simulink model "Urban_Air_Mobility_v3"  (R2021a)
settings: Solver=ode4  StartTime=0.0  StopTime=50  FixedStep=0.01  RelTol=1e-3
model workspace (MAT data in the model file):
  op_trim2 : handle (value not decoded)
undefined symbols (not defined in the file or in its folder): BackProp, Earth, ForwProp, geo, initialise, mass, simsetup, WGS84
libraries: dspindex x6, aerolibactuator x4, sharedutil x3, simulink x3, aerolibasang x2, aerolibtransform2 x2, aerolibutil x2, shared6dof x1, aerolibatmos2 x1, sharedtransform x1, aerolibconvert2 x1
(part 2 of 3)

== system Urban_Air_Mobility_v3/Urban Air Vehicle Airframe Flight Dynamic Model/Lateral Directional Derivatives ==
  Mass (kg) : Inport
  Altitude (m) : Inport  Port=2
  Mach no. : Inport  Port=3
  CG (m) : Inport  Port=4
  CYb : Lookup_n-D  NumberOfTableDimensions=4  BreakpointsForDimension1=initialise.mass  BreakpointsForDimension2=initialise.Altitude  BreakpointsForDimension3=initialise.MLUT  BreakpointsForDimension4=initialise.CG  Table=initialise.CYb  InternalRulePriority=Speed  RndMeth=Simplest  InputSameDT=on
      settings: InputPortMap=u0,u1,u2,u3
  CYp : Lookup_n-D  NumberOfTableDimensions=4  BreakpointsForDimension1=initialise.mass  BreakpointsForDimension2=initialise.Altitude  BreakpointsForDimension3=initialise.MLUT  BreakpointsForDimension4=initialise.CG  Table=initialise.CYp  InternalRulePriority=Speed  RndMeth=Simplest  InputSameDT=on
      settings: InputPortMap=u0,u1,u2,u3
  CYr : Lookup_n-D  NumberOfTableDimensions=4  BreakpointsForDimension1=initialise.mass  BreakpointsForDimension2=initialise.Altitude  BreakpointsForDimension3=initialise.MLUT  BreakpointsForDimension4=initialise.CG  Table=initialise.CYr  InternalRulePriority=Speed  RndMeth=Simplest  InputSameDT=on
      settings: InputPortMap=u0,u1,u2,u3
  Clb : Lookup_n-D  NumberOfTableDimensions=4  BreakpointsForDimension1=initialise.mass  BreakpointsForDimension2=initialise.Altitude  BreakpointsForDimension3=initialise.MLUT  BreakpointsForDimension4=initialise.CG  Table=initialise.Clb  InternalRulePriority=Speed  RndMeth=Simplest  InputSameDT=on
      settings: InputPortMap=u0,u1,u2,u3
  Clp : Lookup_n-D  NumberOfTableDimensions=4  BreakpointsForDimension1=initialise.mass  BreakpointsForDimension2=initialise.Altitude  BreakpointsForDimension3=initialise.MLUT  BreakpointsForDimension4=initialise.CG  Table=initialise.Clp  InternalRulePriority=Speed  RndMeth=Simplest  InputSameDT=on
      settings: InputPortMap=u0,u1,u2,u3
  Clr : Lookup_n-D  NumberOfTableDimensions=4  BreakpointsForDimension1=initialise.mass  BreakpointsForDimension2=initialise.Altitude  BreakpointsForDimension3=initialise.MLUT  BreakpointsForDimension4=initialise.CG  Table=initialise.Clr  InternalRulePriority=Speed  RndMeth=Simplest  InputSameDT=on
      settings: InputPortMap=u0,u1,u2,u3
  "Cnb " : Lookup_n-D  NumberOfTableDimensions=4  BreakpointsForDimension1=initialise.mass  BreakpointsForDimension2=initialise.Altitude  BreakpointsForDimension3=initialise.MLUT  BreakpointsForDimension4=initialise.CG  Table=initialise.Cnb  InternalRulePriority=Speed  RndMeth=Simplest  InputSameDT=on
      settings: InputPortMap=u0,u1,u2,u3
  Cnp : Lookup_n-D  NumberOfTableDimensions=4  BreakpointsForDimension1=initialise.mass  BreakpointsForDimension2=initialise.Altitude  BreakpointsForDimension3=initialise.MLUT  BreakpointsForDimension4=initialise.CG  Table=initialise.Cnp  InternalRulePriority=Speed  RndMeth=Simplest  InputSameDT=on
      settings: InputPortMap=u0,u1,u2,u3
  Cnr : Lookup_n-D  NumberOfTableDimensions=4  BreakpointsForDimension1=initialise.mass  BreakpointsForDimension2=initialise.Altitude  BreakpointsForDimension3=initialise.MLUT  BreakpointsForDimension4=initialise.CG  Table=initialise.Cnr  InternalRulePriority=Speed  RndMeth=Simplest  InputSameDT=on
      settings: InputPortMap=u0,u1,u2,u3
  Cn_p : Outport  VectorParamsAs1DForOutWhenUnconnected=off
  Cn_r : Outport  Port=2  VectorParamsAs1DForOutWhenUnconnected=off
  Cl_p : Outport  Port=3  VectorParamsAs1DForOutWhenUnconnected=off
  Cl_r : Outport  Port=4  VectorParamsAs1DForOutWhenUnconnected=off
  CY_p : Outport  Port=5  VectorParamsAs1DForOutWhenUnconnected=off
  CY_r : Outport  Port=6  VectorParamsAs1DForOutWhenUnconnected=off
  CY_b : Outport  Port=7  VectorParamsAs1DForOutWhenUnconnected=off
  Cl_b : Outport  Port=8  VectorParamsAs1DForOutWhenUnconnected=off
  Cn_b : Outport  Port=9
  wires:
  CG (m)/1 -> Clb/4, CYb/4, "Cnb "/4, CYr/4, CYp/4, Clr/4, Clp/4, Cnr/4, Cnp/4
  Mass (kg)/1 -> Clb/1, CYb/1, "Cnb "/1, CYr/1, CYp/1, Clr/1, Clp/1, Cnr/1, Cnp/1
  Clp/1 -> Cl_p/1
  Cnr/1 -> Cn_r/1
  Cnp/1 -> Cn_p/1
  Mach no./1 -> Clb/3, CYb/3, "Cnb "/3, CYr/3, CYp/3, Clr/3, Clp/3, Cnr/3, Cnp/3
  Clr/1 -> Cl_r/1
  CYr/1 -> CY_r/1
  CYp/1 -> CY_p/1
  CYb/1 -> CY_b/1
  Clb/1 -> Cl_b/1
  Altitude (m)/1 -> Clb/2, CYb/2, "Cnb "/2, CYr/2, CYp/2, Clr/2, Clp/2, Cnr/2, Cnp/2
  "Cnb "/1 -> Cn_b/1

== system Urban_Air_Mobility_v3/Urban Air Vehicle Airframe Flight Dynamic Model/Longitudinal Derivatives ==
  Mass (kg) : Inport
  Altitude (m) : Inport  Port=2
  Mach no. : Inport  Port=3
  CG (m) : Inport  Port=4
  CLalpha : Lookup_n-D  NumberOfTableDimensions=4  BreakpointsForDimension1=initialise.mass  BreakpointsForDimension2=initialise.Altitude  BreakpointsForDimension3=initialise.MLUT  BreakpointsForDimension4=initialise.CG  Table=initialise.CLa  InternalRulePriority=Speed  RndMeth=Simplest  InputSameDT=on
      settings: InputPortMap=u0,u1,u2,u3
  CLq : Lookup_n-D  NumberOfTableDimensions=4  BreakpointsForDimension1=initialise.mass  BreakpointsForDimension2=initialise.Altitude  BreakpointsForDimension3=initialise.MLUT  BreakpointsForDimension4=initialise.CG  Table=initialise.CLq  InternalRulePriority=Speed  RndMeth=Simplest  InputSameDT=on
      settings: InputPortMap=u0,u1,u2,u3
  Cmalpha : Lookup_n-D  NumberOfTableDimensions=4  BreakpointsForDimension1=initialise.mass  BreakpointsForDimension2=initialise.Altitude  BreakpointsForDimension3=initialise.MLUT  BreakpointsForDimension4=initialise.CG  Table=initialise.Cma  InternalRulePriority=Speed  RndMeth=Simplest  InputSameDT=on
      settings: InputPortMap=u0,u1,u2,u3
  Cmq : Lookup_n-D  NumberOfTableDimensions=4  BreakpointsForDimension1=initialise.mass  BreakpointsForDimension2=initialise.Altitude  BreakpointsForDimension3=initialise.MLUT  BreakpointsForDimension4=initialise.CG  Table=initialise.Cmq  InternalRulePriority=Speed  RndMeth=Simplest  InputSameDT=on
      settings: InputPortMap=u0,u1,u2,u3
  CL_alpha : Outport  VectorParamsAs1DForOutWhenUnconnected=off
  CL_q : Outport  Port=2  VectorParamsAs1DForOutWhenUnconnected=off
  Cm_alpha : Outport  Port=3  VectorParamsAs1DForOutWhenUnconnected=off
  Cm_q : Outport  Port=4  VectorParamsAs1DForOutWhenUnconnected=off
  wires:
  CG (m)/1 -> Cmq/4, Cmalpha/4, CLq/4, CLalpha/4
  Mass (kg)/1 -> Cmq/1, Cmalpha/1, CLq/1, CLalpha/1
  Cmalpha/1 -> Cm_alpha/1
  CLq/1 -> CL_q/1
  CLalpha/1 -> CL_alpha/1
  Mach no./1 -> Cmq/3, Cmalpha/3, CLq/3, CLalpha/3
  Cmq/1 -> Cm_q/1
  Altitude (m)/1 -> Cmq/2, Cmalpha/2, CLq/2, CLalpha/2

== system Urban_Air_Mobility_v3/Urban Air Vehicle Airframe Flight Dynamic Model/Zero conditions ==
  Mass (kg) : Inport
  Altitude (m) : Inport  Port=2
  Mach no. : Inport  Port=3
  Re : Inport  Port=4
  CG (m) : Inport  Port=5
  Drag Coefficient CD0 : Lookup_n-D  BreakpointsForDimension1=initialise.Re_range  BreakpointsForDimension2=initialise.Mach_range  BreakpointsForDimension3=initialise.MLUT  BreakpointsForDimension4=initialise.CG  Table=initialise.CD0  InternalRulePriority=Speed  RndMeth=Simplest  InputSameDT=on
      settings: InputPortMap=u0,u1
  Drag Coefficient CM : Lookup_n-D  NumberOfTableDimensions=4  BreakpointsForDimension1=initialise.mass  BreakpointsForDimension2=initialise.Altitude  BreakpointsForDimension3=initialise.MLUT  BreakpointsForDimension4=initialise.CG  Table=initialise.Cm0  InternalRulePriority=Speed  RndMeth=Simplest  InputSameDT=on
      settings: InputPortMap=u0,u1,u2,u3
  Lift Coefficient CL : Lookup_n-D  NumberOfTableDimensions=4  BreakpointsForDimension1=initialise.mass  BreakpointsForDimension2=initialise.Altitude  BreakpointsForDimension3=initialise.MLUT  BreakpointsForDimension4=initialise.CG  Table=initialise.CL0  InternalRulePriority=Speed  RndMeth=Simplest  InputSameDT=on
      settings: InputPortMap=u0,u1,u2,u3
  CL0 : Outport  VectorParamsAs1DForOutWhenUnconnected=off
  CD0 : Outport  Port=2  VectorParamsAs1DForOutWhenUnconnected=off
  CM0 : Outport  Port=3  VectorParamsAs1DForOutWhenUnconnected=off
  wires:
  CG (m)/1 -> Drag Coefficient CM/4, Lift Coefficient CL/4
  Mass (kg)/1 -> Drag Coefficient CM/1, Lift Coefficient CL/1
  Drag Coefficient CD0/1 -> CD0/1
  Lift Coefficient CL/1 -> CL0/1
  Mach no./1 -> Drag Coefficient CM/3, Drag Coefficient CD0/2, Lift Coefficient CL/3
  Altitude (m)/1 -> Drag Coefficient CM/2, Lift Coefficient CL/2
  Drag Coefficient CM/1 -> CM0/1
  Re/1 -> Drag Coefficient CD0/1

== system Urban_Air_Mobility_v3/Urban Air Vehicle Airframe Flight Dynamic Model/Forces and Moments calculation/Ground Effect  ==
  h_above_ground : Inport
  <q_dyn (Pa)> : Inport  Port=2
  CL_alpha : Inport  Port=3
  Drag : Inport  Port=4
  Lift : Inport  Port=5
  CL_dF : Inport  Port=6
  Cm_dF : Inport  Port=7
  Flap : Inport  Port=8
  VTAS : Inport  Port=9
  Enable : EnablePort  StatesWhenEnabling=reset
  Constant3 : Constant  Value=geo.mac_w
  Constant5 : Constant  Value=geo.b_fus+geo.b_w
  Constant6 : Constant  Value=geo.b_fus+geo.b_w
  Constant7 : Constant  Value=geo.S_w
  Constant8 : Constant  Value=geo.S_w
  Divide : Product  Inputs=*/
  Ground : Ground
  MATLAB Function1 : MATLAB Function  TreatAsAtomicUnit=on
  Square : Math  Operator=square  SignedPower=on  SaturateOnIntegerOverflow=on
  "Delta_lift " : Outport  OutputWhenDisabled=reset  InitialOutput=[0]  VectorParamsAs1DForOutWhenUnconnected=off
  Delta_drag : Outport  Port=2  OutputWhenDisabled=reset  InitialOutput=[0]  VectorParamsAs1DForOutWhenUnconnected=off
  Delta_CL : Outport  Port=3  OutputWhenDisabled=reset  InitialOutput=[0]  VectorParamsAs1DForOutWhenUnconnected=off
  "Delta_CD " : Outport  Port=4  OutputWhenDisabled=reset  InitialOutput=[0]  VectorParamsAs1DForOutWhenUnconnected=off
  wires:
  Constant8/1 -> MATLAB Function1/13(S_ref)
  MATLAB Function1/4(delta_Drag) -> Delta_drag/1
  MATLAB Function1/3(delta_Lift) -> "Delta_lift "/1
  Square/1 -> Divide/1
  Constant7/1 -> Divide/2
  Constant6/1 -> Square/1
  Divide/1 -> [C]
  CL_dF/1 -> MATLAB Function1/8(CL_dF)
  Lift/1 -> MATLAB Function1/7(Lift)
  CL_alpha/1 -> MATLAB Function1/1(lift_curve_slope)
  Constant3/1 -> MATLAB Function1/3(c_bar)
  h_above_ground/1 -> MATLAB Function1/2(height_above_ground)
  Cm_dF/1 -> MATLAB Function1/9(Cm_dF)
  Ground/1 -> MATLAB Function1/11(wing_thickness)
  [C] -> MATLAB Function1/5(AR)
  Drag/1 -> MATLAB Function1/6(Drag)
  Constant5/1 -> MATLAB Function1/4(b)
  <q_dyn (Pa)>/1 -> MATLAB Function1/12(q_dyn)
  MATLAB Function1/1(delta_CL) -> Delta_CL/1
  MATLAB Function1/2(delta_CD) -> "Delta_CD "/1
  Flap/1 -> MATLAB Function1/10(Flap)
  VTAS/1 -> MATLAB Function1/14(VTAS)

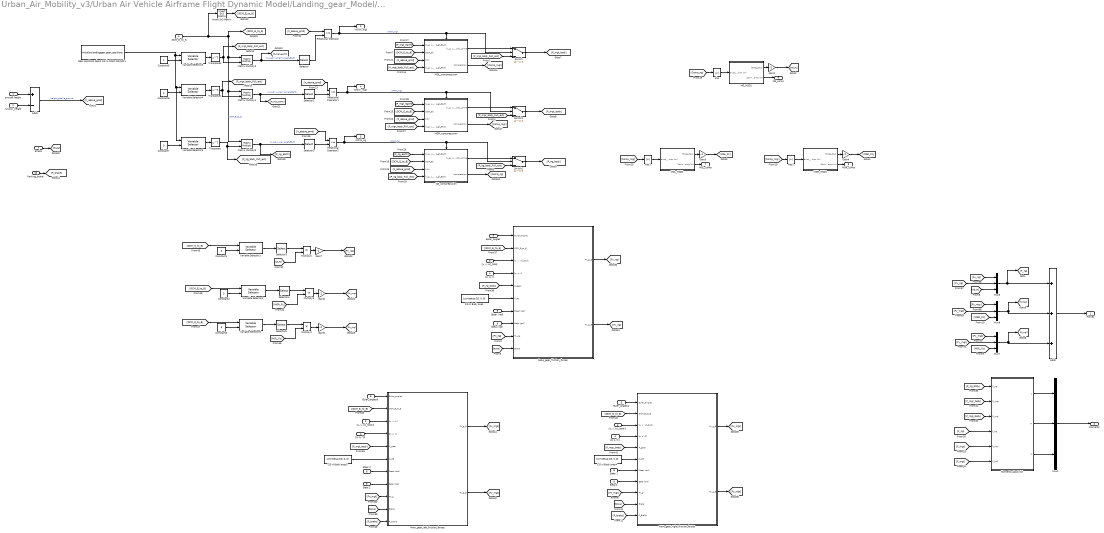
== system Urban_Air_Mobility_v3/Urban Air Vehicle Airframe Flight Dynamic Model/Landing_gear_Model/Landing Gear (with steer 4) ==
  aircraft height : Inport
  runway_height : Inport  Port=2
  DCM_B_to_E : Inport  Port=3
  "[p, q, r]" : Inport  Port=4
  "[u, v, w]_body" : Inport  Port=5
  Euler_angles : Inport  Port=6
  "Brake " : Inport  Port=7
  "Steer (rad) " : Inport  Port=8
  "Beta (rad) " : Inport  Port=9
  Parking_brake : Inport  Port=10
  Abs : Abs
  Abs1 : Abs
  Abs2 : Abs
  Add1 : Sum  Inputs=+-
  Add2 : Sum  Inputs=+++
  Beta 1 : InportShadow  Port=9
  Beta 2 : InportShadow  Port=9
  CG in Body axes : Constant  Value=[simsetup.CG, 0, 0]
  CG in Body axes3 : Constant  Value=[simsetup.CG, 0, 0]
  CG in Body axes4 : Constant  Value=[simsetup.CG, 0, 0]
  Constant{1..3,7} (4 alike) : Constant  Value=3
  Constant5 : Constant
  Constant6 : Constant  Value=2
  Euler_angles2 : InportShadow  Port=6
  Euler_angles6 : InportShadow  Port=6
  Gain{2..4,7..9} (6 alike) : Gain  Gain=-1
  Gear positions about CG (L.MG;R.MG;NG)1 : Constant  Value=initialise.landinggear.gear_positions
  Invert 3x3 Matrix : aerolibutil/Invert  3x3 Matrix
  MGL_MSD1 : Subsystem
  MGL_compresssion : Subsystem
  MGR_MSD1 : Subsystem
  MGR_compresssion : Subsystem
  Main_gear_left_friction_forces : Subsystem
  Main_gear_right_friction_forces : Subsystem
  Matrix Multiply3 : Product  Multiplication=Matrix(*)
  Matrix Multiply4 : Product  Multiplication=Matrix(*)
  Matrix Multiply5 : Product  Multiplication=Matrix(*)
  Moments about CG : MATLAB Function  TreatAsAtomicUnit=on
  Multiply2 : Product
  Multiply3 : Product
  Multiply4 : Product
  Mux{1,6..8} (4 alike) : Mux  Inputs=3
  NG_MSD1 : Subsystem
  NG_compresssion : Subsystem
  Nose_gear_friction_forces : Subsystem
  Relational Operator : RelationalOperator  Operator=<=  OutDataTypeStr=boolean  RndMeth=Simplest
  Relational Operator1 : RelationalOperator  Operator=<=  OutDataTypeStr=boolean  RndMeth=Simplest
  Relational Operator2 : RelationalOperator  Operator=<=  OutDataTypeStr=boolean  RndMeth=Simplest
  Selector{,1..5} (6 alike) : Selector  InputPortWidth=3  IndexOptions=Index vector (dialog)  Indices=3  OutputSizes=1
  Steer 1 : InportShadow  Port=8
  Steer 2 : InportShadow  Port=8
  Switch : Switch  Criteria=u2 ~= 0
  Switch1 : Switch  Criteria=u2 ~= 0
  Switch2 : Switch  Criteria=u2 ~= 0
  Transpose : Math  Operator=transpose  SignedPower=on  SaturateOnIntegerOverflow=on
  Transpose1 : Math  Operator=transpose  SignedPower=on  SaturateOnIntegerOverflow=on
  Transpose2 : Math  Operator=transpose  SignedPower=on  SaturateOnIntegerOverflow=on
  Variable Selector{1..6} (6 alike) : dspindex/Variable Selector  NumInputs=1  rowsOrCols=Rows  IdxMode=Variable  Elements=[1 3]  ZerOneIdxMode=One-based  errmode=Clip Index  FillMode=on  FillValues=0
  "[p, q, r]1" : InportShadow  Port=4
  "[p, q, r]2" : InportShadow  Port=4
  "[u, v, w]_body1" : InportShadow  Port=5
  "[u, v, w]_body2" : InportShadow  Port=5
  "Forces " : Outport  VectorParamsAs1DForOutWhenUnconnected=off
  Moments : Outport  Port=2  VectorParamsAs1DForOutWhenUnconnected=off
  WOW_mgl : Outport  Port=3  VectorParamsAs1DForOutWhenUnconnected=off
  WOW_mglr : Outport  Port=4  VectorParamsAs1DForOutWhenUnconnected=off
  "WOW_ng " : Outport  Port=5  VectorParamsAs1DForOutWhenUnconnected=off
  NG_comp : Outport  Port=6  VectorParamsAs1DForOutWhenUnconnected=off
  MGL_comp : Outport  Port=7  VectorParamsAs1DForOutWhenUnconnected=off
  MGR_comp : Outport  Port=8  VectorParamsAs1DForOutWhenUnconnected=off
  wires:
  Constant7/1 -> Variable Selector5/2
  [Fy_mgr] -> Mux8/2
  Selector2/1 -> Relational Operator2/2
  Selector/1 -> Relational Operator/2
  MGR_MSD1/1(Force_strut) -> Gain4/1
  DCM_B_to_E/1 -> Matrix Multiply5/1, Matrix Multiply4/1, Matrix Multiply3/1, [DCM_B_to_E], Invert 3x3 Matrix/1  "DCM_B_to_E"
  [Fx_mgr] -> Mux8/1
  MGL_compresssion/1("[x_g, y_g, z_g]_Body_prime") -> Switch/1
  Mux8/1 -> [F_mgr], Add2/2
  Relational Operator1/1 -> MGR_compresssion/Enable, Switch1/2, WOW_mglr/1  "WOW_mgr"
  [MGL_Fz] -> Mux7/3
  Gain4/1 -> [MGR_Fz]
  [P_mgl_body_Full_ext] -> MGL_compresssion/4("[x_g, y_g, z_g]_Body")
  [Comp_ng] -> Abs/1
  [Fy_ng] -> Mux6/2
  [DCM_E_to_B] -> NG_compresssion/2("DCM_eb ")
  [Fx_ng] -> Mux6/1
  [NG_Fz] -> Mux6/3
  [DCM_E_to_B] -> MGL_compresssion/2("DCM_eb ")
  [Comp_mgl] -> Abs1/1
  Matrix Multiply3/1 -> [P_mgl_earth], Selector/1  "[x_mgl, y_mgl, z_mgl]_Earth"
  Constant5/1 -> Variable Selector3/2
  MGL_MSD1/1(Force_strut) -> Gain3/1
  [MGR_Fz] -> Mux8/3
  [Fx_mgl] -> Mux7/1
  Add2/1 -> "Forces "/1
  Constant6/1 -> Variable Selector4/2
  [Fy_mgl] -> Mux7/2
  Variable Selector4/1 -> Transpose1/1
  Add1/1 -> [h_above_grnd]  "height_above_ground"
  Variable Selector3/1 -> Transpose2/1
  Variable Selector5/1 -> Transpose/1
  MGL_MSD1/2(Spring_comp (m)) -> MGL_comp/1
  Mux6/1 -> [F_ng], Add2/1
  [DCM_E_to_B] -> MGR_compresssion/2("DCM_eb ")
  Relational Operator/1 -> WOW_mgl/1, Switch/2, MGL_compresssion/Enable  "WOW_mgl"
  Mux7/1 -> [F_mgl], Add2/3
  Matrix Multiply4/1 -> [P_mgr_earth], Selector1/1  "[x_mgr, y_mgr, z_mgr]_Earth"
  Gain3/1 -> [MGL_Fz]
  [Comp_mgr] -> Abs2/1
  Selector1/1 -> Relational Operator1/2
  NG_MSD1/1(Force_strut) -> Gain2/1
  MGR_MSD1/2(Spring_comp (m)) -> MGR_comp/1
  [P_ng_body_Full_ext] -> NG_compresssion/4("[x_g, y_g, z_g]_Body")
  MGR_compresssion/2(compression) -> [Comp_mgr]
  NG_MSD1/2(Spring_comp (m)) -> NG_comp/1
  Gain2/1 -> [NG_Fz]
  Matrix Multiply5/1 -> [P_ng_earth], Selector2/1  "[x_ng, y_ng, z_ng]_Earth"
  NG_compresssion/2(compression) -> [Comp_ng]
  Relational Operator2/1 -> NG_compresssion/Enable, Switch2/2, "WOW_ng "/1  "WOW_ng"
  Invert 3x3 Matrix/1 -> [DCM_E_to_B]
  [P_mgr_body_Full_ext] -> MGR_compresssion/4("[x_g, y_g, z_g]_Body")
  NG_compresssion/1("[x_g, y_g, z_g]_Body_prime") -> Switch2/1
  runway_height/1 -> Add1/2
  MGR_compresssion/1("[x_g, y_g, z_g]_Body_prime") -> Switch1/1
  aircraft height/1 -> Add1/1
  [P_mgl_body_Full_ext] -> Switch/3
  Switch/1 -> [P_mgl_body]
  [P_mgr_body_Full_ext] -> Switch1/3
  Switch1/1 -> [P_mgr_body]
  [P_ng_body_Full_ext] -> Switch2/3
  Switch2/1 -> [P_ng_body]
  MGL_compresssion/2(compression) -> [Comp_mgl]
  Abs/1 -> NG_MSD1/1("axial_deflection (m) ")
  Abs1/1 -> MGL_MSD1/1("axial_deflection (m) ")
  Abs2/1 -> MGR_MSD1/1("axial_deflection (m) ")
  Transpose/1 -> [P_ng_body_Full_ext], Matrix Multiply5/2
  Transpose1/1 -> Matrix Multiply4/2, [P_mgr_body_Full_ext]
  Transpose2/1 -> Matrix Multiply3/2, [P_mgl_body_Full_ext]
  [h_above_grnd] -> MGL_compresssion/3("h-hr ")
  [h_above_grnd] -> MGR_compresssion/3("h-hr ")
  [h_above_grnd] -> NG_compresssion/3("h-hr ")
  [h_above_grnd] -> Relational Operator/1
  [h_above_grnd] -> Relational Operator1/1
  [h_above_grnd] -> Relational Operator2/1
  [P_mgl_earth] -> MGL_compresssion/1("[x_g, y_g, z_g]_Earth")
  [P_mgr_earth] -> MGR_compresssion/1("[x_g, y_g, z_g]_Earth")
  [P_ng_earth] -> NG_compresssion/1("[x_g, y_g, z_g]_Earth")
  [F_mgr] -> Moments about CG/5(F_mgr)
  [F_ng] -> Moments about CG/4(F_ng)
  Moments about CG/1(L) -> Mux1/1
  Mux1/1 -> Moments/1
  [F_mgl] -> Moments about CG/6(F_mgl)
  Moments about CG/3(N) -> Mux1/3
  [P_mgl_body] -> Moments about CG/3(P_mgl)
  Moments about CG/2(M) -> Mux1/2
  [P_ng_body] -> Moments about CG/1(P_ng)
  [P_mgr_body] -> Moments about CG/2(P_mgr)
  Gear positions about CG (L.MG;R.MG;NG)1/1 -> Variable Selector5/1, Variable Selector4/1, Variable Selector3/1
  [DCM_E_to_B] -> Variable Selector1/1
  Constant1/1 -> Variable Selector1/2
  Variable Selector1/1 -> Selector3/1
  Selector3/1 -> Multiply2/1
  [NG_Fz] -> Multiply2/2
  Multiply2/1 -> Gain7/1
  Multiply3/1 -> Gain8/1
  [MGR_Fz] -> Multiply3/2
  Selector4/1 -> Multiply3/1
  Variable Selector2/1 -> Selector4/1
  Constant2/1 -> Variable Selector2/2
  [DCM_E_to_B] -> Variable Selector2/1
  [DCM_E_to_B] -> Variable Selector6/1
  Constant3/1 -> Variable Selector6/2
  Variable Selector6/1 -> Selector5/1
  Selector5/1 -> Multiply4/1
  [MGL_Fz] -> Multiply4/2
  Multiply4/1 -> Gain9/1
  Gain7/1 -> [Fn_ng]
  Gain8/1 -> [Fn_mgr]
  Gain9/1 -> [Fn_mgl]
  "Brake "/1 -> [Brake]
  Parking_brake/1 -> [P_brake]
  Euler_angles/1 -> Nose_gear_friction_forces/1(Euler_angles)
  [DCM_B_to_E] -> Nose_gear_friction_forces/2(DCM_B_to_E)
  "[u, v, w]_body"/1 -> Nose_gear_friction_forces/3("[u, v, w]_body")
  "[p, q, r]"/1 -> Nose_gear_friction_forces/4("[p, q, r]")
  [P_ng_body] -> Nose_gear_friction_forces/5(P_gear)
  CG in Body axes/1 -> Nose_gear_friction_forces/6(P_cg)
  "Steer (rad) "/1 -> Nose_gear_friction_forces/7("Steer (rad) ")
  "Beta (rad) "/1 -> Nose_gear_friction_forces/8("Beta (rad) ")
  Nose_gear_friction_forces/1(Fx_g_E) -> [Fx_ng]
  Nose_gear_friction_forces/2(Fy_g_E) -> [Fy_ng]
  [Fn_ng] -> Nose_gear_friction_forces/9(Fn_ng)
  [Brake] -> Nose_gear_friction_forces/10("Brake ")
  [DCM_B_to_E] -> Main_gear_right_friction_forces/2(DCM_B_to_E)
  "[u, v, w]_body1"/1 -> Main_gear_right_friction_forces/3("[u, v, w]_body")
  "[p, q, r]1"/1 -> Main_gear_right_friction_forces/4("[p, q, r]]")
  [P_mgr_body] -> Main_gear_right_friction_forces/5(P_gear)
  Beta 1/1 -> Main_gear_right_friction_forces/8("Beta (rad) ")
  CG in Body axes4/1 -> Main_gear_right_friction_forces/6(P_CG)
  Steer 1/1 -> Main_gear_right_friction_forces/7("Steer (rad) ")
  Euler_angles2/1 -> Main_gear_right_friction_forces/1(Euler_angles)
  Main_gear_right_friction_forces/1(Fx_g_E) -> [Fx_mgr]
  Main_gear_right_friction_forces/2(Fy_g_E) -> [Fy_mgr]
  [Fn_mgr] -> Main_gear_right_friction_forces/9(Fn_g)
  [P_brake] -> Main_gear_right_friction_forces/11(P_Brake)
  [Brake] -> Main_gear_right_friction_forces/10(Brake)
  Euler_angles6/1 -> Main_gear_left_friction_forces/1(Euler_angles)
  [DCM_B_to_E] -> Main_gear_left_friction_forces/2(DCM_B_to_E)
  "[u, v, w]_body2"/1 -> Main_gear_left_friction_forces/3("[u, v, w]")
  "[p, q, r]2"/1 -> Main_gear_left_friction_forces/4("[p, q, r]")
  [P_mgl_body] -> Main_gear_left_friction_forces/5(P_gear)
  Beta 2/1 -> Main_gear_left_friction_forces/8("Beta (rad) ")
  CG in Body axes3/1 -> Main_gear_left_friction_forces/6(P_CG)
  Steer 2/1 -> Main_gear_left_friction_forces/7("Steer (rad) ")
  Main_gear_left_friction_forces/1(Fx_g_E) -> [Fx_mgl]
  Main_gear_left_friction_forces/2(Fy_g_E) -> [Fy_mgl]
  [Brake] -> Main_gear_left_friction_forces/10(Brake)
  [Fn_mgl] -> Main_gear_left_friction_forces/9(Fn_g)
  [P_brake] -> Main_gear_left_friction_forces/11(P_brake)

== system Urban_Air_Mobility_v3/Urban Air Vehicle Airframe Flight Dynamic Model/Landing_gear_Model/UC Aero Forces and Moments ==
  alpha : Inport
  Re : Inport  Port=2
  q_dyn : Inport  Port=3
  beta : Inport  Port=4
  flap_d : Inport  Port=5
  Angle Conversion : aerolibconvert2/Angle Conversion  IU=rad  OU=deg
  CD_main_landing_gear : Lookup_n-D  NumberOfTableDimensions=3  BreakpointsForDimension1=initialise.landinggear.aero.re  BreakpointsForDimension2=initialise.landinggear.aero.alpha  BreakpointsForDimension3=initialise.landinggear.aero.dflap  BreakpointsForDimension4=initialise.CG  Table=initialise.landinggear.aero.CD_maingear  InternalRulePriority=Speed  RndMeth=Simplest  InputSameDT=on
      settings: InputPortMap=u0,u1,u2
  CD_main_landing_gear to calculate side force : Lookup_n-D  NumberOfTableDimensions=3  BreakpointsForDimension1=initialise.landinggear.aero.re  BreakpointsForDimension2=initialise.landinggear.aero.alpha  BreakpointsForDimension3=initialise.landinggear.aero.dflap  BreakpointsForDimension4=initialise.CG  Table=initialise.landinggear.aero.CD_maingear  InternalRulePriority=Speed  RndMeth=Simplest  InputSameDT=on
      settings: InputPortMap=u0,u1,u2
  CD_nose_landing_gear : Lookup_n-D  BreakpointsForDimension1=initialise.landinggear.aero.re  BreakpointsForDimension2=initialise.landinggear.aero.alpha  BreakpointsForDimension3=initialise.landingear.dflap  BreakpointsForDimension4=initialise.CG  Table=initialise.landinggear.aero.CD_nosegear  InternalRulePriority=Speed  RndMeth=Simplest  InputSameDT=on
      settings: InputPortMap=u0,u1
  CD_nose_landing_gear to calculate side force : Lookup_n-D  BreakpointsForDimension1=initialise.landinggear.aero.re  BreakpointsForDimension2=initialise.landinggear.aero.alpha  BreakpointsForDimension3=initialise.landingear.dflap  BreakpointsForDimension4=initialise.CG  Table=initialise.landinggear.aero.CD_nosegear  InternalRulePriority=Speed  RndMeth=Simplest  InputSameDT=on
      settings: InputPortMap=u0,u1
  Constant1 : Constant  Value=0
  Gear positions about CG (L.MG;R.MG;NG)1 : Constant  Value=initialise.landinggear.gear_positions
  MATLAB Function : MATLAB Function  TreatAsAtomicUnit=on
  alpha1 : InportShadow
  z_main_landing_gear : Lookup_n-D  BreakpointsForDimension1=initialise.landinggear.aero.re  BreakpointsForDimension2=initialise.landinggear.aero.alpha  BreakpointsForDimension3=initialise.landingear.dflap  BreakpointsForDimension4=initialise.CG  Table=initialise.landinggear.aero.z_maingear  InternalRulePriority=Speed  RndMeth=Simplest  InputSameDT=on
      settings: InputPortMap=u0,u1
  z_nose_landing_gear : Lookup_n-D  BreakpointsForDimension1=initialise.landinggear.aero.re  BreakpointsForDimension2=initialise.landinggear.aero.alpha  BreakpointsForDimension3=initialise.landingear.dflap  BreakpointsForDimension4=initialise.CG  Table=initialise.landinggear.aero.z_nosegear  InternalRulePriority=Speed  RndMeth=Simplest  InputSameDT=on
      settings: InputPortMap=u0,u1
  UC_aero_forces : Outport  VectorParamsAs1DForOutWhenUnconnected=off
  wires:
  alpha/1 -> Angle Conversion/1  "alpha"
  Re/1 -> z_nose_landing_gear/1, z_main_landing_gear/1, CD_nose_landing_gear to calculate side force/1, CD_main_landing_gear to calculate side force/1, CD_nose_landing_gear/1, CD_main_landing_gear/1  "Re"
  q_dyn/1 -> MATLAB Function/1(q_dyn)  "q"
  flap_d/1 -> CD_main_landing_gear/3  "flap_d"
  z_main_landing_gear/1 -> MATLAB Function/8(z_mg)
  z_nose_landing_gear/1 -> MATLAB Function/9(z_ng)  "z_nosegear"
  Angle Conversion/1 -> z_nose_landing_gear/2, z_main_landing_gear/2, CD_main_landing_gear to calculate side force/3, CD_nose_landing_gear/2, CD_main_landing_gear/2
  Constant1/1 -> CD_nose_landing_gear to calculate side force/2, CD_main_landing_gear to calculate side force/2
  alpha1/1 -> MATLAB Function/2(alpha)  "alpha"
  beta/1 -> MATLAB Function/3(beta)  "beta"
  CD_main_landing_gear/1 -> MATLAB Function/4(CD_mg)
  CD_nose_landing_gear/1 -> MATLAB Function/5(CD_ng)
  CD_main_landing_gear to calculate side force/1 -> MATLAB Function/6(dfy_mg)
  CD_nose_landing_gear to calculate side force/1 -> MATLAB Function/7(dfy_ng)
  Gear positions about CG (L.MG;R.MG;NG)1/1 -> MATLAB Function/10(UC_pos)
  MATLAB Function/1(UC_forces) -> UC_aero_forces/1

== system Urban_Air_Mobility_v3/Urban Air Vehicle Airframe Flight Dynamic Model/Landing_gear_Model/Landing Gear (with steer 4)/MGL_MSD1 ==
  "axial_deflection (m) " : Inport
  Add : Sum
  Derivative : Derivative
  Stiffness : Gain  Gain=initialise.landinggear.K
  Viscous Damping : Gain  Gain=initialise.landinggear.C
  deflection_range_limit : Saturate  UpperLimit=1.5  LowerLimit=0
  Force_strut : Outport  VectorParamsAs1DForOutWhenUnconnected=off
  Spring_comp (m) : Outport  Port=2  VectorParamsAs1DForOutWhenUnconnected=off
  wires:
  "axial_deflection (m) "/1 -> deflection_range_limit/1
  Add/1 -> Force_strut/1  "Force_strut"
  Stiffness/1 -> Add/1
  deflection_range_limit/1 -> Spring_comp (m)/1, Derivative/1, Stiffness/1
  Derivative/1 -> Viscous Damping/1
  Viscous Damping/1 -> Add/2

== system Urban_Air_Mobility_v3/Urban Air Vehicle Airframe Flight Dynamic Model/Landing_gear_Model/Landing Gear (with steer 4)/MGL_compresssion ==
  "[x_g, y_g, z_g]_Earth" : Inport
  "DCM_eb " : Inport  Port=2
  "h-hr " : Inport  Port=3
  "[x_g, y_g, z_g]_Body" : Inport  Port=4
  Enable : EnablePort  StatesWhenEnabling=reset
  Demux : Demux  Outputs=3
  Matrix Multiply1 : Product  Multiplication=Matrix(*)
  Mux : Mux  Inputs=3
  Scope : Scope
  Selector3 : Selector  InputPortWidth=3  IndexOptions=Index vector (dialog)  Indices=3  OutputSizes=1
  Selector4 : Selector  InputPortWidth=3  IndexOptions=Index vector (dialog)  Indices=3  OutputSizes=1
  Subtract2 : Sum  Inputs=+-
  Terminator : Terminator
  "[x_g, y_g, z_g]_Body_prime" : Outport  VectorParamsAs1DForOutWhenUnconnected=off
  compression : Outport  Port=2  OutputWhenDisabled=reset  InitialOutput=[0]  VectorParamsAs1DForOutWhenUnconnected=off
  wires:
  "DCM_eb "/1 -> Matrix Multiply1/1
  Demux/2 -> Mux/2
  Demux/1 -> Mux/1
  Mux/1 -> Matrix Multiply1/2
  Matrix Multiply1/1 -> Selector3/1, "[x_g, y_g, z_g]_Body_prime"/1
  "[x_g, y_g, z_g]_Earth"/1 -> Demux/1
  Subtract2/1 -> Scope/1, compression/1  "comp"
  Selector3/1 -> Subtract2/2
  Selector4/1 -> Subtract2/1
  "[x_g, y_g, z_g]_Body"/1 -> Selector4/1
  Demux/3 -> Terminator/1
  "h-hr "/1 -> Mux/3

== system Urban_Air_Mobility_v3/Urban Air Vehicle Airframe Flight Dynamic Model/Landing_gear_Model/Landing Gear (with steer 4)/MGR_MSD1 ==
  "axial_deflection (m) " : Inport
  Add : Sum
  Derivative : Derivative
  Stiffness : Gain  Gain=initialise.landinggear.K
  Viscous Damping : Gain  Gain=initialise.landinggear.C
  deflection_range_limit : Saturate  UpperLimit=1.5  LowerLimit=0
  Force_strut : Outport  VectorParamsAs1DForOutWhenUnconnected=off
  Spring_comp (m) : Outport  Port=2  VectorParamsAs1DForOutWhenUnconnected=off
  wires:
  Viscous Damping/1 -> Add/2
  Derivative/1 -> Viscous Damping/1
  deflection_range_limit/1 -> Stiffness/1, Derivative/1, Spring_comp (m)/1
  Stiffness/1 -> Add/1
  Add/1 -> Force_strut/1  "Force_strut"
  "axial_deflection (m) "/1 -> deflection_range_limit/1

== system Urban_Air_Mobility_v3/Urban Air Vehicle Airframe Flight Dynamic Model/Landing_gear_Model/Landing Gear (with steer 4)/MGR_compresssion ==
  "[x_g, y_g, z_g]_Earth" : Inport
  "DCM_eb " : Inport  Port=2
  "h-hr " : Inport  Port=3
  "[x_g, y_g, z_g]_Body" : Inport  Port=4
  Enable : EnablePort  StatesWhenEnabling=reset
  Demux : Demux  Outputs=3
  Matrix Multiply1 : Product  Multiplication=Matrix(*)
  Mux : Mux  Inputs=3
  Selector3 : Selector  InputPortWidth=3  IndexOptions=Index vector (dialog)  Indices=3  OutputSizes=1
  Selector4 : Selector  InputPortWidth=3  IndexOptions=Index vector (dialog)  Indices=3  OutputSizes=1
  Subtract2 : Sum  Inputs=+-
  Terminator : Terminator
  "[x_g, y_g, z_g]_Body_prime" : Outport  VectorParamsAs1DForOutWhenUnconnected=off
  compression : Outport  Port=2  OutputWhenDisabled=reset  InitialOutput=[0]  VectorParamsAs1DForOutWhenUnconnected=off
  wires:
  "[x_g, y_g, z_g]_Body"/1 -> Selector4/1
  Selector4/1 -> Subtract2/1
  Selector3/1 -> Subtract2/2
  Subtract2/1 -> compression/1  "comp"
  "[x_g, y_g, z_g]_Earth"/1 -> Demux/1
  Matrix Multiply1/1 -> "[x_g, y_g, z_g]_Body_prime"/1, Selector3/1
  Mux/1 -> Matrix Multiply1/2
  Demux/1 -> Mux/1
  "h-hr "/1 -> Mux/3
  Demux/2 -> Mux/2
  Demux/3 -> Terminator/1
  "DCM_eb "/1 -> Matrix Multiply1/1

== system Urban_Air_Mobility_v3/Urban Air Vehicle Airframe Flight Dynamic Model/Landing_gear_Model/Landing Gear (with steer 4)/Main_gear_left_friction_forces ==
  Euler_angles : Inport
  DCM_B_to_E : Inport  Port=2
  "[u, v, w]" : Inport  Port=3
  "[p, q, r]" : Inport  Port=4
  P_gear : Inport  Port=5
  P_CG : Inport  Port=6
  "Steer (rad) " : Inport  Port=7
  "Beta (rad) " : Inport  Port=8
  Fn_g : Inport  Port=9
  Brake : Inport  Port=10
  P_brake : Inport  Port=11
  Euler_angles1 : InportShadow
  GP to Earth axes 2 : Subsystem
  MGL_friction_forces : Subsystem
  Velocity at MGL in ground path : Subsystem
  Fx_g_E : Outport  VectorParamsAs1DForOutWhenUnconnected=off
  Fy_g_E : Outport  Port=2  VectorParamsAs1DForOutWhenUnconnected=off
  wires:
  Velocity at MGL in ground path/2(v_g_gp) -> [v_mgl_gp]
  GP to Earth axes 2/2(Fy_g_E) -> Fy_g_E/1
  Brake/1 -> MGL_friction_forces/4(Brake)
  Velocity at MGL in ground path/1(u_g_gp) -> [u_mgl_gp]
  [F_long_mgl] -> GP to Earth axes 2/2(F_long_g)
  Euler_angles1/1 -> Velocity at MGL in ground path/6(Euler)
  [v_mgl_gp] -> MGL_friction_forces/3(v_gp)
  MGL_friction_forces/1(F_g_long) -> [F_long_mgl]
  Euler_angles/1 -> GP to Earth axes 2/1(Euler Angles)
  "[p, q, r]"/1 -> Velocity at MGL in ground path/3("[p, q, r]")
  [F_lat_mgl] -> GP to Earth axes 2/3(F_lat_g)
  [u_mgl_gp] -> MGL_friction_forces/2(u_gp)
  MGL_friction_forces/2(F_g_lat) -> [F_lat_mgl]
  "Beta (rad) "/1 -> MGL_friction_forces/5("Beta ")
  "Steer (rad) "/1 -> MGL_friction_forces/6(Steer 1)
  P_brake/1 -> MGL_friction_forces/7(P_brake)
  GP to Earth axes 2/1(Fx_g_E) -> Fx_g_E/1
  P_gear/1 -> Velocity at MGL in ground path/4(P_gear)
  "[u, v, w]"/1 -> Velocity at MGL in ground path/2(V_b)
  DCM_B_to_E/1 -> Velocity at MGL in ground path/1(DCM_B_to_E)
  P_CG/1 -> Velocity at MGL in ground path/5(P_cg)
  Fn_g/1 -> MGL_friction_forces/1("Fn_g ")

== system Urban_Air_Mobility_v3/Urban Air Vehicle Airframe Flight Dynamic Model/Landing_gear_Model/Landing Gear (with steer 4)/Main_gear_right_friction_forces ==
  Euler_angles : Inport
  DCM_B_to_E : Inport  Port=2
  "[u, v, w]_body" : Inport  Port=3
  "[p, q, r]]" : Inport  Port=4
  P_gear : Inport  Port=5
  P_CG : Inport  Port=6
  "Steer (rad) " : Inport  Port=7
  "Beta (rad) " : Inport  Port=8
  Fn_g : Inport  Port=9
  Brake : Inport  Port=10
  P_Brake : Inport  Port=11
  Euler_angles1 : InportShadow
  GP to Earth axes 1 : Subsystem
  MGR_friction_forces : Subsystem
  Velocity at MGR in ground path : Subsystem
  Fx_g_E : Outport  VectorParamsAs1DForOutWhenUnconnected=off
  Fy_g_E : Outport  Port=2  VectorParamsAs1DForOutWhenUnconnected=off
  wires:
  "Beta (rad) "/1 -> MGR_friction_forces/5("Beta ")
  P_gear/1 -> Velocity at MGR in ground path/4(P_gear)
  MGR_friction_forces/1(F_g_long) -> [F_long_mgr]
  [F_long_mgr] -> GP to Earth axes 1/2(F_long_g)
  P_Brake/1 -> MGR_friction_forces/7(P_brake)
  Velocity at MGR in ground path/1(u_g_gp) -> [u_mgr_gp]
  Velocity at MGR in ground path/2(v_g_gp) -> [v_mgr_gp]
  Euler_angles1/1 -> GP to Earth axes 1/1(Euler Angles)
  [u_mgr_gp] -> MGR_friction_forces/2(u_gp)
  MGR_friction_forces/2(F_g_lat) -> [F_lat_mgr]
  [F_lat_mgr] -> GP to Earth axes 1/3(F_lat_g)
  [v_mgr_gp] -> MGR_friction_forces/3(v_gp)
  "Steer (rad) "/1 -> MGR_friction_forces/6("steer ")
  Euler_angles/1 -> Velocity at MGR in ground path/6(Euler)
  GP to Earth axes 1/2(Fy_g_E) -> Fy_g_E/1
  DCM_B_to_E/1 -> Velocity at MGR in ground path/1(DCM_B_to_E)
  P_CG/1 -> Velocity at MGR in ground path/5(P_cg)
  "[p, q, r]]"/1 -> Velocity at MGR in ground path/3("[p, q, r]")
  Fn_g/1 -> MGR_friction_forces/1("Fn_g ")
  Brake/1 -> MGR_friction_forces/4(Brake)
  "[u, v, w]_body"/1 -> Velocity at MGR in ground path/2(V_b)
  GP to Earth axes 1/1(Fx_g_E) -> Fx_g_E/1

== system Urban_Air_Mobility_v3/Urban Air Vehicle Airframe Flight Dynamic Model/Landing_gear_Model/Landing Gear (with steer 4)/NG_MSD1 ==
  "axial_deflection (m) " : Inport
  Add : Sum
  Derivative : Derivative
  Stiffness : Gain  Gain=initialise.landinggear.K
  Viscous Damping : Gain  Gain=initialise.landinggear.C
  deflection_range_limit : Saturate  UpperLimit=1.5  LowerLimit=0
  Force_strut : Outport  VectorParamsAs1DForOutWhenUnconnected=off
  Spring_comp (m) : Outport  Port=2  VectorParamsAs1DForOutWhenUnconnected=off
  wires:
  Viscous Damping/1 -> Add/2
  Derivative/1 -> Viscous Damping/1
  deflection_range_limit/1 -> Stiffness/1, Derivative/1, Spring_comp (m)/1
  Stiffness/1 -> Add/1
  Add/1 -> Force_strut/1  "Force_strut"
  "axial_deflection (m) "/1 -> deflection_range_limit/1

== system Urban_Air_Mobility_v3/Urban Air Vehicle Airframe Flight Dynamic Model/Landing_gear_Model/Landing Gear (with steer 4)/NG_compresssion ==
  "[x_g, y_g, z_g]_Earth" : Inport
  "DCM_eb " : Inport  Port=2
  "h-hr " : Inport  Port=3
  "[x_g, y_g, z_g]_Body" : Inport  Port=4
  Enable : EnablePort  StatesWhenEnabling=reset
  Demux : Demux  Outputs=3
  Matrix Multiply1 : Product  Multiplication=Matrix(*)
  Mux : Mux  Inputs=3
  Selector3 : Selector  InputPortWidth=3  IndexOptions=Index vector (dialog)  Indices=3  OutputSizes=1
  Selector4 : Selector  InputPortWidth=3  IndexOptions=Index vector (dialog)  Indices=3  OutputSizes=1
  Subtract2 : Sum  Inputs=+-
  Terminator : Terminator
  "[x_g, y_g, z_g]_Body_prime" : Outport  VectorParamsAs1DForOutWhenUnconnected=off
  compression : Outport  Port=2  OutputWhenDisabled=reset  InitialOutput=[0]  VectorParamsAs1DForOutWhenUnconnected=off
  wires:
  "DCM_eb "/1 -> Matrix Multiply1/1
  Demux/3 -> Terminator/1
  Demux/2 -> Mux/2
  "h-hr "/1 -> Mux/3
  Demux/1 -> Mux/1
  Mux/1 -> Matrix Multiply1/2
  Matrix Multiply1/1 -> Selector3/1, "[x_g, y_g, z_g]_Body_prime"/1
  "[x_g, y_g, z_g]_Earth"/1 -> Demux/1
  Subtract2/1 -> compression/1  "comp"
  Selector3/1 -> Subtract2/2
  Selector4/1 -> Subtract2/1
  "[x_g, y_g, z_g]_Body"/1 -> Selector4/1

== system Urban_Air_Mobility_v3/Urban Air Vehicle Airframe Flight Dynamic Model/Landing_gear_Model/Landing Gear (with steer 4)/Nose_gear_friction_forces ==
  Euler_angles : Inport
  DCM_B_to_E : Inport  Port=2
  "[u, v, w]_body" : Inport  Port=3
  "[p, q, r]" : Inport  Port=4
  P_gear : Inport  Port=5
  P_cg : Inport  Port=6
  "Steer (rad) " : Inport  Port=7
  "Beta (rad) " : Inport  Port=8
  Fn_ng : Inport  Port=9
  "Brake " : Inport  Port=10
  Euler_angles1 : InportShadow
  "GP to Earth axes " : Subsystem
  NG_friction_forces : Subsystem
  Steer (rad) _1 : InportShadow  Port=7
  Steer (rad) _2 : InportShadow  Port=7
  Velocity at NG in ground path : Subsystem
  Fx_g_E : Outport  VectorParamsAs1DForOutWhenUnconnected=off
  Fy_g_E : Outport  Port=2  VectorParamsAs1DForOutWhenUnconnected=off
  wires:
  "Beta (rad) "/1 -> NG_friction_forces/6("Beta (rad) ")
  "GP to Earth axes "/1(Fx_g_E) -> Fx_g_E/1
  NG_friction_forces/2(F_g_lat) -> [F_lat_ng]
  P_gear/1 -> Velocity at NG in ground path/4(P_gear)
  [u_ng_gp] -> NG_friction_forces/2(u_gp)
  Steer (rad) _1/1 -> "GP to Earth axes "/4(nose_wheel_angle (rad))
  Velocity at NG in ground path/2(v_g_gp) -> [v_ng_gp]
  "Brake "/1 -> NG_friction_forces/4(Brake)
  Fn_ng/1 -> NG_friction_forces/1("Fn_ng ")
  [F_long_ng] -> "GP to Earth axes "/2(F_long_g)
  [F_lat_ng] -> "GP to Earth axes "/3(F_lat_g)
  [v_ng_gp] -> NG_friction_forces/3(v_gp)
  NG_friction_forces/1(F_g_long) -> [F_long_ng]
  Velocity at NG in ground path/1(u_g_gp) -> [u_ng_gp]
  Euler_angles/1 -> "GP to Earth axes "/1(Euler Angles)
  "Steer (rad) "/1 -> NG_friction_forces/5("Steering (rad) ")
  P_cg/1 -> Velocity at NG in ground path/5(P_cg)
  DCM_B_to_E/1 -> Velocity at NG in ground path/1(DCM_B_to_E)
  "[u, v, w]_body"/1 -> Velocity at NG in ground path/2(V_b)
  "[p, q, r]"/1 -> Velocity at NG in ground path/3("[p, q, r]")
  Euler_angles1/1 -> Velocity at NG in ground path/6(Euler)
  "GP to Earth axes "/2(Fy_g_E) -> Fy_g_E/1
  Steer (rad) _2/1 -> Velocity at NG in ground path/7("nose_wheel_steering (rad) ")

== system Urban_Air_Mobility_v3/Urban Air Vehicle Airframe Flight Dynamic Model/Landing_gear_Model/Landing Gear (with steer 4)/Main_gear_left_friction_forces/GP to Earth axes 2 ==
  Euler Angles : Inport
  F_long_g : Inport  Port=2
  F_lat_g : Inport  Port=3
  Multiply{9..12} (4 alike) : Product
  Selector6 : Selector  InputPortWidth=3  IndexOptions=Index vector (dialog)  Indices=3  OutputSizes=1
  Sin : Trigonometry
  Sin1 : Trigonometry  Operator=cos
  Subtract : Sum  Inputs=+-
  Subtract1 : Sum
  Fx_g_E : Outport  VectorParamsAs1DForOutWhenUnconnected=off
  Fy_g_E : Outport  Port=2  VectorParamsAs1DForOutWhenUnconnected=off
  wires:
  Sin1/1 -> [cos_psi]
  [cos_psi] -> Multiply9/2
  Euler Angles/1 -> Selector6/1
  Multiply10/1 -> Subtract/2
  Sin/1 -> [sin_psi]
  Multiply12/1 -> Subtract1/1
  F_lat_g/1 -> Multiply11/1, Multiply10/2
  F_long_g/1 -> Multiply9/1, Multiply12/1
  Subtract1/1 -> Fy_g_E/1  "Fy_g_E"
  Subtract/1 -> Fx_g_E/1  "Fx_g_E"
  [sin_psi] -> Multiply10/1
  [sin_psi] -> Multiply12/2
  [cos_psi] -> Multiply11/2
  Multiply11/1 -> Subtract1/2
  Multiply9/1 -> Subtract/1
  Selector6/1 -> Sin/1, Sin1/1  "psi"

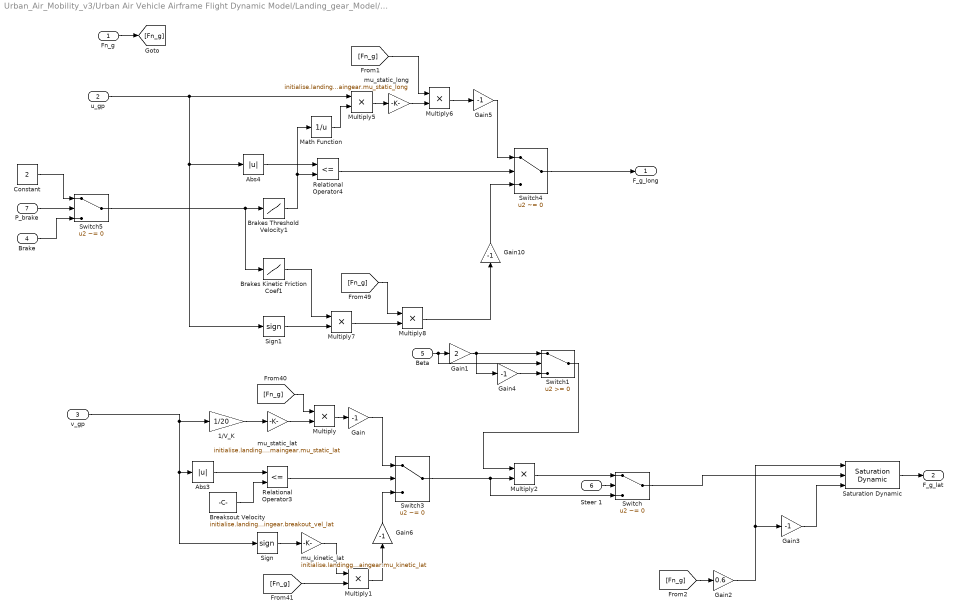
== system Urban_Air_Mobility_v3/Urban Air Vehicle Airframe Flight Dynamic Model/Landing_gear_Model/Landing Gear (with steer 4)/Main_gear_left_friction_forces/MGL_friction_forces ==
  "Fn_g " : Inport
  u_gp : Inport  Port=2
  v_gp : Inport  Port=3
  Brake : Inport  Port=4
  "Beta " : Inport  Port=5
  Steer 1 : Inport  Port=6
  P_brake : Inport  Port=7
  1/V_K : Gain  Gain=1/20
  Abs3 : Abs
  Abs4 : Abs
  Brakes Kinetic Friction Coef1 : Lookup  InputValues=[0 1 2]  Table=[0.1 0.5 0.8]
  Brakes Threshold Velocity1 : Lookup  InputValues=[0 1 2]  Table=[0.5, 0.04, 0.04]
  Breaksout Velocity : Constant  Value=initialise.landinggear.maingear.breakout_vel_lat
  Constant : Constant  Value=2
  Gain{,3..6,10} (6 alike) : Gain  Gain=-1
  Gain1 : Gain  Gain=2
  Gain2 : Gain  Gain=0.6
  Math Function : Math  Operator=reciprocal  SignedPower=on  SaturateOnIntegerOverflow=on
  Multiply{,1..2,5..8} (7 alike) : Product
  Relational Operator3 : RelationalOperator  Operator=<=  OutDataTypeStr=boolean  RndMeth=Simplest
  Relational Operator4 : RelationalOperator  Operator=<=  OutDataTypeStr=boolean  RndMeth=Simplest
  Saturation Dynamic : simulink/Discontinuities/Saturation Dynamic  OutMin=[]  OutMax=[]  OutDataTypeStr=Inherit: Same as second input  OutDataType=fixdt(1, 16)  OutScaling=2^-10  DoSatur=off
  Sign : Signum
  Sign1 : Signum
  Switch{,3..5} (4 alike) : Switch  Criteria=u2 ~= 0
  Switch1 : Switch
  mu_kinetic_lat : Gain  Gain=initialise.landinggear.maingear.mu_kinetic_lat
  mu_static_lat : Gain  Gain=initialise.landinggear.maingear.mu_static_lat
  mu_static_long : Gain  Gain=initialise.landinggear.maingear.mu_static_long
  F_g_long : Outport  VectorParamsAs1DForOutWhenUnconnected=off
  F_g_lat : Outport  Port=2  VectorParamsAs1DForOutWhenUnconnected=off
  wires:
  Multiply1/1 -> Gain6/1
  Switch4/1 -> F_g_long/1
  Math Function/1 -> Multiply5/2
  Abs4/1 -> Relational Operator4/1
  Sign1/1 -> Multiply7/2
  Multiply5/1 -> mu_static_long/1
  u_gp/1 -> Multiply5/1, Sign1/1, Abs4/1
  Multiply6/1 -> Gain5/1
  Brakes Threshold Velocity1/1 -> Relational Operator4/2, Math Function/1
  Multiply8/1 -> Gain10/1
  Multiply7/1 -> Multiply8/2
  [Fn_g] -> Multiply8/1
  mu_static_lat/1 -> Multiply/2
  Multiply/1 -> Gain/1
  Relational Operator4/1 -> Switch4/2
  Gain5/1 -> Switch4/1
  mu_static_long/1 -> Multiply6/2
  v_gp/1 -> 1/V_K/1, Sign/1, Abs3/1
  mu_kinetic_lat/1 -> Multiply1/1
  Gain10/1 -> Switch4/3
  Abs3/1 -> Relational Operator3/1
  [Fn_g] -> Multiply/1
  Sign/1 -> mu_kinetic_lat/1
  1/V_K/1 -> mu_static_lat/1
  Relational Operator3/1 -> Switch3/2
  Gain/1 -> Switch3/1
  Breaksout Velocity/1 -> Relational Operator3/2
  Brakes Kinetic Friction Coef1/1 -> Multiply7/1
  Gain6/1 -> Switch3/3
  "Fn_g "/1 -> [Fn_g]
  [Fn_g] -> Multiply6/1
  Switch3/1 -> Switch/3, Multiply2/2
  Saturation Dynamic/1 -> F_g_lat/1
  [Fn_g] -> Multiply1/2
  [Fn_g] -> Gain2/1
  Gain2/1 -> Gain3/1, Saturation Dynamic/1
  Gain3/1 -> Saturation Dynamic/3
  Multiply2/1 -> Switch/1
  Switch/1 -> Saturation Dynamic/2
  Steer 1/1 -> Switch/2
  Gain1/1 -> Gain4/1, Switch1/1
  "Beta "/1 -> Switch1/2, Gain1/1
  Gain4/1 -> Switch1/3
  Switch1/1 -> Multiply2/1
  Switch5/1 -> Brakes Kinetic Friction Coef1/1, Brakes Threshold Velocity1/1
  Brake/1 -> Switch5/3
  P_brake/1 -> Switch5/2
  Constant/1 -> Switch5/1

== system Urban_Air_Mobility_v3/Urban Air Vehicle Airframe Flight Dynamic Model/Landing_gear_Model/Landing Gear (with steer 4)/Main_gear_left_friction_forces/Velocity at MGL in ground path ==
  DCM_B_to_E : Inport
  V_b : Inport  Port=2
  "[p, q, r]" : Inport  Port=3
  P_gear : Inport  Port=4
  P_cg : Inport  Port=5
  Euler : Inport  Port=6
  Demux : Demux  Outputs=3
  Ground Path Velocities : Subsystem
  Matrix Multiply1 : Product  Multiplication=Matrix(*)
  Mux2 : Mux  Inputs=3
  Velocity at gear in body axes : MATLAB Function  TreatAsAtomicUnit=on
  u_g_gp : Outport  VectorParamsAs1DForOutWhenUnconnected=off
  v_g_gp : Outport  Port=2  VectorParamsAs1DForOutWhenUnconnected=off
  wires:
  Demux/1 -> Velocity at gear in body axes/2(p)
  Demux/3 -> Velocity at gear in body axes/4(r)
  DCM_B_to_E/1 -> Matrix Multiply1/1
  Velocity at gear in body axes/2(v_g) -> Mux2/2
  Matrix Multiply1/1 -> Ground Path Velocities/1(V_ng_earth)  "V_ng_earth"
  Velocity at gear in body axes/1(u_g) -> Mux2/1
  Mux2/1 -> Matrix Multiply1/2  "[u_ng, v_ng, w_ng]_body"
  Velocity at gear in body axes/3(w_g) -> Mux2/3
  Demux/2 -> Velocity at gear in body axes/3(q)
  P_gear/1 -> Velocity at gear in body axes/5(P_g)
  V_b/1 -> Velocity at gear in body axes/1(V_b)
  "[p, q, r]"/1 -> Demux/1
  Ground Path Velocities/1(u_ng_ground_path) -> u_g_gp/1
  Euler/1 -> Ground Path Velocities/2("Euler ")
  Ground Path Velocities/2(v_ng_ground_path) -> v_g_gp/1
  P_cg/1 -> Velocity at gear in body axes/6(P_cg)

== system Urban_Air_Mobility_v3/Urban Air Vehicle Airframe Flight Dynamic Model/Landing_gear_Model/Landing Gear (with steer 4)/Main_gear_right_friction_forces/GP to Earth axes 1 ==
  Euler Angles : Inport
  F_long_g : Inport  Port=2
  F_lat_g : Inport  Port=3
  Display5 : Display
  Display6 : Display
  Multiply{9..12} (4 alike) : Product
  Scope : Scope
  Scope5 : Scope
  Selector6 : Selector  InputPortWidth=3  IndexOptions=Index vector (dialog)  Indices=3  OutputSizes=1
  Sin : Trigonometry
  Sin1 : Trigonometry  Operator=cos
  Subtract : Sum  Inputs=+-
  Subtract1 : Sum
  Fx_g_E : Outport  VectorParamsAs1DForOutWhenUnconnected=off
  Fy_g_E : Outport  Port=2  VectorParamsAs1DForOutWhenUnconnected=off
  wires:
  Multiply9/1 -> Subtract/1
  Multiply11/1 -> Subtract1/2
  [cos_psi] -> Multiply11/2
  [sin_psi] -> Multiply12/2
  [sin_psi] -> Multiply10/1
  Subtract/1 -> Scope/1, Fx_g_E/1, Display5/1  "Fx_g_E"
  Subtract1/1 -> Scope5/1, Fy_g_E/1, Display6/1  "Fy_g_E"
  F_long_g/1 -> Multiply12/1, Multiply9/1
  F_lat_g/1 -> Multiply10/2, Multiply11/1
  Multiply12/1 -> Subtract1/1
  Sin/1 -> [sin_psi]
  Multiply10/1 -> Subtract/2
  Euler Angles/1 -> Selector6/1
  [cos_psi] -> Multiply9/2
  Sin1/1 -> [cos_psi]
  Selector6/1 -> Sin/1, Sin1/1  "psi"

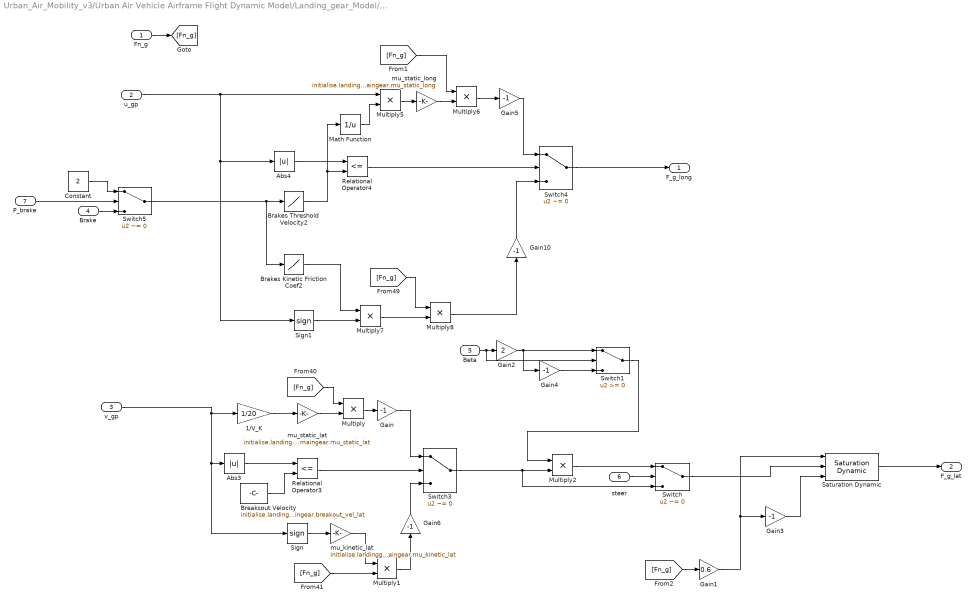
== system Urban_Air_Mobility_v3/Urban Air Vehicle Airframe Flight Dynamic Model/Landing_gear_Model/Landing Gear (with steer 4)/Main_gear_right_friction_forces/MGR_friction_forces ==
  "Fn_g " : Inport
  u_gp : Inport  Port=2
  v_gp : Inport  Port=3
  Brake : Inport  Port=4
  "Beta " : Inport  Port=5
  "steer " : Inport  Port=6
  P_brake : Inport  Port=7
  1/V_K : Gain  Gain=1/20
  Abs3 : Abs
  Abs4 : Abs
  Brakes Kinetic Friction Coef2 : Lookup  InputValues=[0 1 2]  Table=[0.1 0.5 0.8]
  Brakes Threshold Velocity2 : Lookup  InputValues=[0 1 2]  Table=[0.5, 0.04, 0.04]
  Breaksout Velocity : Constant  Value=initialise.landinggear.maingear.breakout_vel_lat
  Constant : Constant  Value=2
  Gain{,3..6,10} (6 alike) : Gain  Gain=-1
  Gain1 : Gain  Gain=0.6
  Gain2 : Gain  Gain=2
  Math Function : Math  Operator=reciprocal  SignedPower=on  SaturateOnIntegerOverflow=on
  Multiply{,1..2,5..8} (7 alike) : Product
  Relational Operator3 : RelationalOperator  Operator=<=  OutDataTypeStr=boolean  RndMeth=Simplest
  Relational Operator4 : RelationalOperator  Operator=<=  OutDataTypeStr=boolean  RndMeth=Simplest
  Saturation Dynamic : simulink/Discontinuities/Saturation Dynamic  OutMin=[]  OutMax=[]  OutDataTypeStr=Inherit: Same as second input  OutDataType=fixdt(1, 16)  OutScaling=2^-10  DoSatur=off
  Sign : Signum
  Sign1 : Signum
  Switch{,3..5} (4 alike) : Switch  Criteria=u2 ~= 0
  Switch1 : Switch
  mu_kinetic_lat : Gain  Gain=initialise.landinggear.maingear.mu_kinetic_lat
  mu_static_lat : Gain  Gain=initialise.landinggear.maingear.mu_static_lat
  mu_static_long : Gain  Gain=initialise.landinggear.maingear.mu_static_long
  F_g_long : Outport  VectorParamsAs1DForOutWhenUnconnected=off
  F_g_lat : Outport  Port=2  VectorParamsAs1DForOutWhenUnconnected=off
  wires:
  [Fn_g] -> Multiply6/1
  "Fn_g "/1 -> [Fn_g]
  Gain6/1 -> Switch3/3
  [Fn_g] -> Multiply1/2
  Brakes Kinetic Friction Coef2/1 -> Multiply7/1
  Breaksout Velocity/1 -> Relational Operator3/2
  Gain/1 -> Switch3/1
  Relational Operator3/1 -> Switch3/2
  1/V_K/1 -> mu_static_lat/1
  Sign/1 -> mu_kinetic_lat/1
  [Fn_g] -> Multiply/1
  Abs3/1 -> Relational Operator3/1
  Gain10/1 -> Switch4/3
  mu_kinetic_lat/1 -> Multiply1/1
  v_gp/1 -> 1/V_K/1, Abs3/1, Sign/1
  mu_static_long/1 -> Multiply6/2
  Gain5/1 -> Switch4/1
  Relational Operator4/1 -> Switch4/2
  Multiply/1 -> Gain/1
  mu_static_lat/1 -> Multiply/2
  [Fn_g] -> Multiply8/1
  Multiply7/1 -> Multiply8/2
  Multiply8/1 -> Gain10/1
  Brakes Threshold Velocity2/1 -> Math Function/1, Relational Operator4/2
  Multiply6/1 -> Gain5/1
  u_gp/1 -> Abs4/1, Sign1/1, Multiply5/1
  Multiply5/1 -> mu_static_long/1
  Sign1/1 -> Multiply7/2
  Abs4/1 -> Relational Operator4/1
  Math Function/1 -> Multiply5/2
  Switch4/1 -> F_g_long/1
  Multiply1/1 -> Gain6/1
  Switch3/1 -> Switch/3, Multiply2/2
  "Beta "/1 -> Switch1/2, Gain2/1
  Gain3/1 -> Saturation Dynamic/3
  Gain1/1 -> Gain3/1, Saturation Dynamic/1
  [Fn_g] -> Gain1/1
  Saturation Dynamic/1 -> F_g_lat/1
  Gain2/1 -> Gain4/1, Switch1/1
  Multiply2/1 -> Switch/1
  "steer "/1 -> Switch/2
  Switch/1 -> Saturation Dynamic/2
  Gain4/1 -> Switch1/3
  Switch1/1 -> Multiply2/1
  Switch5/1 -> Brakes Kinetic Friction Coef2/1, Brakes Threshold Velocity2/1
  Brake/1 -> Switch5/3
  P_brake/1 -> Switch5/2
  Constant/1 -> Switch5/1
